simulink model "part1"  (R2023a)
settings: Solver=ode4  StartTime=0.0  StopTime=100  FixedStep=0.01  RelTol=1e-3
values from neighbouring files (symbols this model uses):
  Af = diag ([1/t1, 1/t2, 1/t3])    [init.m]
  Gamma_Matrix = diag(omega.^2)    [init.m]
  Kd = [2030000 5950000 763500000]    [init.m]
  Ki = [1586 23000 1068000]    [init.m]
  Kp = [114000 788000 78300000]    [init.m]
  Omega_Matrix = diag (2*zeta.*omega)    [init.m]
  P0 = eye(15)    [CPM.m]
  Q = eye(6)    [CPM.m]    (also in control_plant_model.m)
  R = eye(3)    [CPM.m]    (also in control_plant_model.m)
  ref_model = 1    [init.m]    (also in plotter.m; sim1.m; sim2.m; sim2_faulty.m)
  sample_time = 0.1    [CPM.m]    (also in init.m = 0.01)
  simulation = 4    [init.m]    (also in plotter.m)
  x0 = zeros(15,1)    [CPM.m]
undefined symbols (not defined in the file or in its folder): Hoerner, model, thrusters, vessel
libraries: eeStairGenerator x6, simulink x3, marine_gnc x3, slpidlib x3, marine_hydro x2
settings Model: Creator=jonbjor  LastModifiedBy=33769
settings SolverCC: AlgebraicLoopSolver=TrustRegion
settings DataIOCC: ReturnWorkspaceOutputs=off
settings DebuggingCC: UnconnectedInputMsg=warning  UnconnectedOutputMsg=warning  UnconnectedLineMsg=warning  ArithmeticOperatorsInVariantConditions=warning
settings ModelReferenceCC: EnableRefExpFcnMdlSchedulingChecks=on
settings SFSimCC: SimUseLocalCustomCode=off  CustomCodeUndefinedFunction=UseInterfaceOnly
settings RTWCC: RTWUseLocalCustomCode=off  DLArmComputeVersion=19.05

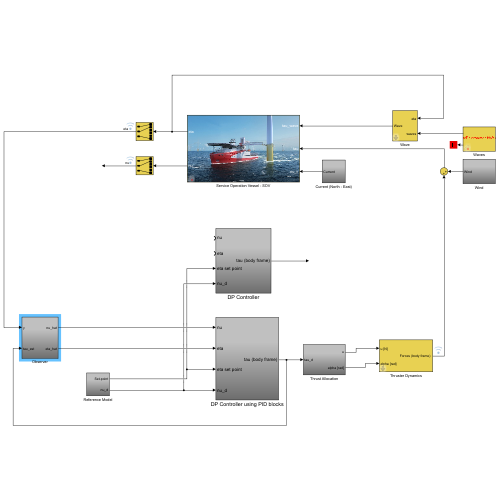
[thumbnail: Simulink's stored preview of the top-level diagram]
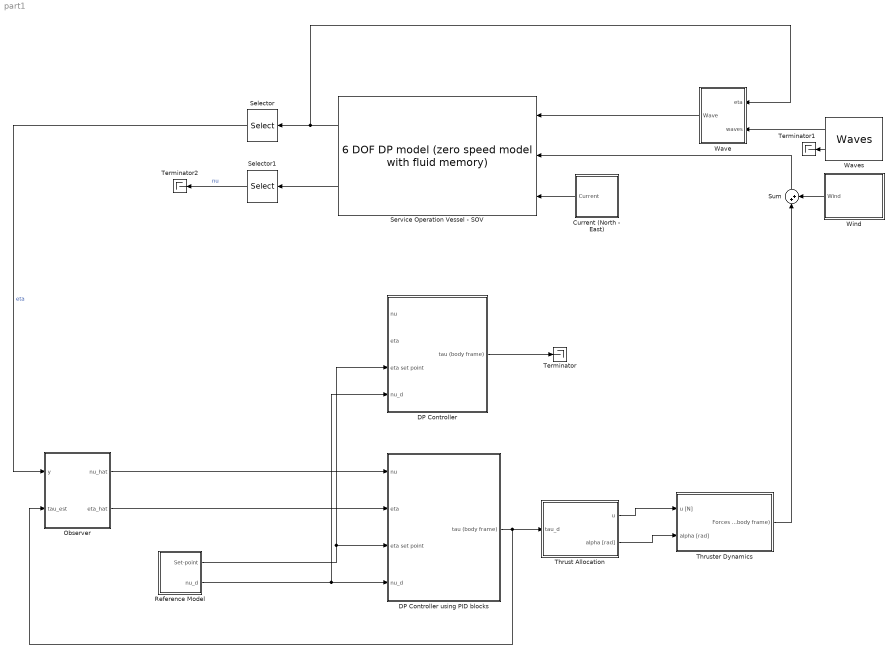
== system part1 ==
  Current (North - East) : Subsystem
  DP Controller : Subsystem
  DP Controller using PID blocks : Subsystem
  Observer : Subsystem
  Reference Model : Subsystem
  Selector : Selector  InputPortWidth=6  IndexOptions=Index vector (dialog)  Indices=[1 2 6]  OutputSizes=1
  Selector1 : Selector  InputPortWidth=6  IndexOptions=Index vector (dialog)  Indices=[1 2 6]  OutputSizes=1
  Service Operation Vessel - SOV : marine_hydro/Hydro Library/6 DOF DP model  (zero speed model with fluid memory)  ABC=vesselABC  rho=1025  Axc=0.9*vessel.main.T*vessel.main.B  Ayc=0.9*vessel.main.T*vessel.main.Lpp  CX=1  CY_2D=Hoerner(vessel.main.B,vessel.main.T)  Bv=vessel.Bv  mask(6 DOF zero speed model){}
      link override "Integrator1 ": InitialCondition=nu0
      link override Integrator2: InitialCondition=eta0
      mask Display:
      | image('SOV.jpg');
      | color('white'); port_label('output', 1, 'eta')
      | color('white'); port_label('output', 2, 'nu')
      | color('white'); port_label('input', 1, 'tau_wave')
      | color('white'); port_label('input', 2, 'tau')
      | color('white'); port_label('input', 3, 'nu_c')
  Sum : Sum  Inputs=|++
  Terminator : Terminator
  Terminator1 : Terminator
  Terminator2 : Terminator
  Thrust Allocation : Subsystem
  Thruster Dynamics : Subsystem  mask{thrusterfault=off}
      mask prompts: thrusterfault "Fault on thruster #2 and #4?"
  Wave : Subsystem  mask{waveforces=on}
      mask prompts: waveforces "Waveforces enabled"
  Waves : marine_gnc/Environment/Waves/Waves  spectrum_type=ITTC  disp_flag=on  plot_spectrum=off  plot_realization=off  hs=5  omega_peak=pi/10  psi_mean=0  gamma=-1  spread=2  depth=inf  nfreq=20  ndir=10  energylim=0.005  freq_cutoff=3  dir_cutoff=0  rand_seed=123  rand_freq=on  rand_dir=on  Zeta_a=0  Omega=0  Phase=0  Wavenum=0  Psi=0
  Wind : Subsystem
  wires:
  Current (North - East)/1(Current) -> Service Operation Vessel - SOV/3
  Service Operation Vessel - SOV/2 -> Selector1/1
  Selector/1 -> Observer/1(y)  "eta"
  Wave/1(Wave) -> Service Operation Vessel - SOV/1
  Reference Model/1(Set-point) -> DP Controller/3(eta set point), DP Controller using PID blocks/3(eta set point)
  Reference Model/2(nu_d) -> DP Controller/4(nu_d), DP Controller using PID blocks/4(nu_d)
  DP Controller/1(tau (body frame)) -> Terminator/1
  Waves/2 -> Terminator1/1
  Thruster Dynamics/1("Forces (body frame) ") -> Sum/1
  Service Operation Vessel - SOV/1 -> Wave/1(eta), Selector/1
  Wind/1(Wind) -> Sum/2
  Waves/1 -> Wave/2(waves)
  Sum/1 -> Service Operation Vessel - SOV/2
  Thrust Allocation/1(u) -> Thruster Dynamics/1(u [N])
  Thrust Allocation/2(alpha [rad]) -> Thruster Dynamics/2(alpha [rad])
  DP Controller using PID blocks/1(tau (body frame)) -> Observer/2(tau_est), Thrust Allocation/1(tau_d)
  Selector1/1 -> Terminator2/1  "nu"
  Observer/1(nu_hat) -> DP Controller using PID blocks/1(nu)
  Observer/2(eta_hat) -> DP Controller using PID blocks/2(eta)

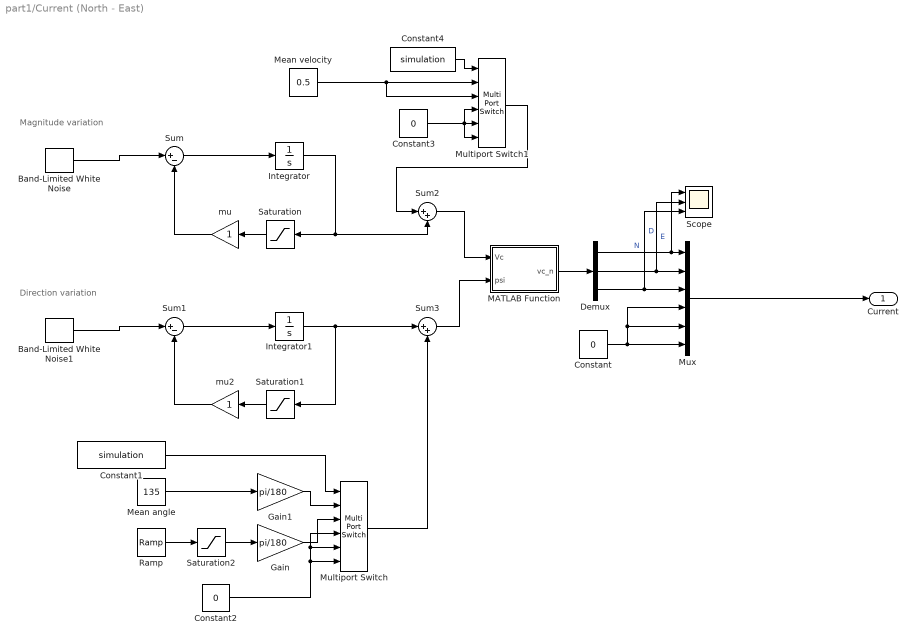
== system part1/Current (North - East) ==
  note: Magnitude variation
  note: Direction variation
  Band-Limited White Noise : simulink/Sources/Band-Limited White Noise  Cov=[0]  Ts=0.1  seed=[23341]
  Band-Limited White Noise1 : simulink/Sources/Band-Limited White Noise  Cov=[0]  Ts=0.1  seed=[23341]
  Constant : Constant  Value=0
  Constant1 : Constant  Value=simulation
  Constant2 : Constant  Value=0
  Constant3 : Constant  Value=0
  Constant4 : Constant  Value=simulation
  Demux : Demux  Outputs=3
  Gain : Gain  Gain=pi/180
  Gain1 : Gain  Gain=pi/180
  Integrator : Integrator
  Integrator1 : Integrator
  MATLAB Function : MATLAB Function  TreatAsAtomicUnit=on
  Mean angle : Constant  Value=135
  Mean velocity : Constant  Value=0.5
  Multiport Switch : MultiPortSwitch  Inputs=4  DataPortForDefault=Additional data port  SaturateOnIntegerOverflow=off  InputSameDT=off
  Multiport Switch1 : MultiPortSwitch  Inputs=4  DataPortForDefault=Additional data port  SaturateOnIntegerOverflow=off  InputSameDT=off
  Mux : Mux  Inputs=6
  Ramp : simulink/Sources/Ramp  slope=1  start=10  InitialOutput=180
  Saturation : Saturate  UpperLimit=1  LowerLimit=0
  Saturation1 : Saturate  UpperLimit=pi  LowerLimit=0
  Saturation2 : Saturate  UpperLimit=270  LowerLimit=0
  Scope : Scope  NumInputPorts=3
  Sum : Sum  Inputs=|+-
  Sum1 : Sum  Inputs=|+-
  Sum2 : Sum  Inputs=|++
  Sum3 : Sum  Inputs=|++
  mu : Gain
  mu2 : Gain
  Current : Outport  VectorParamsAs1DForOutWhenUnconnected=off
  wires:
  Band-Limited White Noise1/1 -> Sum1/1
  Mean velocity/1 -> Multiport Switch1/3, Multiport Switch1/2
  Mean angle/1 -> Gain1/1
  Saturation1/1 -> mu2/1
  Sum/1 -> Integrator/1
  Saturation2/1 -> Gain/1
  mu/1 -> Sum/2
  Constant3/1 -> Multiport Switch1/4, Multiport Switch1/6, Multiport Switch1/5
  Ramp/1 -> Saturation2/1
  Constant2/1 -> Multiport Switch/6, Multiport Switch/5, Multiport Switch/4
  Integrator1/1 -> Saturation1/1, Sum3/1
  Sum3/1 -> MATLAB Function/2(psi)
  Integrator/1 -> Sum2/2, Saturation/1
  Sum2/1 -> MATLAB Function/1(Vc)
  Multiport Switch1/1 -> Sum2/1
  MATLAB Function/1(vc_n) -> Demux/1
  Demux/1 -> Scope/1, Mux/1  "N"
  Constant/1 -> Mux/6, Mux/5, Mux/4
  mu2/1 -> Sum1/2
  Saturation/1 -> mu/1
  Demux/3 -> Scope/3, Mux/3  "D"
  Demux/2 -> Scope/2, Mux/2  "E"
  Gain/1 -> Multiport Switch/3
  Constant1/1 -> Multiport Switch/1
  Gain1/1 -> Multiport Switch/2
  Multiport Switch/1 -> Sum3/2
  Band-Limited White Noise/1 -> Sum/1
  Sum1/1 -> Integrator1/1
  Constant4/1 -> Multiport Switch1/1
  Mux/1 -> Current/1

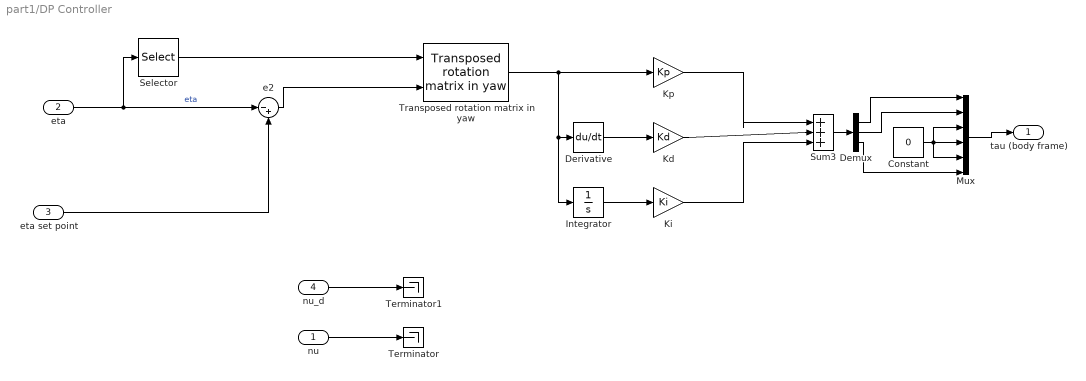
== system part1/DP Controller ==
  nu : Inport
  eta : Inport  Port=2
  eta set point : Inport  Port=3
  nu_d : Inport  Port=4
  Constant : Constant  Value=0
  Demux : Demux  Outputs=3
  Derivative : Derivative
  Integrator : Integrator
  Kd : Gain  Gain=Kd
  Ki : Gain  Gain=Ki
  Kp : Gain  Gain=Kp
  Mux : Mux  Inputs=6
  Selector : Selector  InputPortWidth=3  IndexOptions=Index vector (dialog)  Indices=3  OutputSizes=1
  Sum3 : Sum  Inputs=|+++
  Terminator : Terminator
  Terminator1 : Terminator
  Transposed rotation matrix in yaw : marine_gnc/Models/ Kinematics/Transposed rotation  matrix in yaw
  e2 : Sum  Inputs=|-+
  tau (body frame) : Outport  VectorParamsAs1DForOutWhenUnconnected=off
  wires:
  nu/1 -> Terminator/1
  e2/1 -> Transposed rotation matrix in yaw/2
  Transposed rotation matrix in yaw/1 -> Integrator/1, Derivative/1, Kp/1
  Kp/1 -> Sum3/1
  Derivative/1 -> Kd/1
  Kd/1 -> Sum3/2
  Integrator/1 -> Ki/1
  Ki/1 -> Sum3/3
  nu_d/1 -> Terminator1/1
  eta/1 -> Selector/1, e2/1  "eta"
  eta set point/1 -> e2/2
  Selector/1 -> Transposed rotation matrix in yaw/1
  Sum3/1 -> Demux/1
  Mux/1 -> tau (body frame)/1
  Demux/1 -> Mux/1
  Demux/2 -> Mux/2
  Demux/3 -> Mux/6
  Constant/1 -> Mux/5, Mux/4, Mux/3

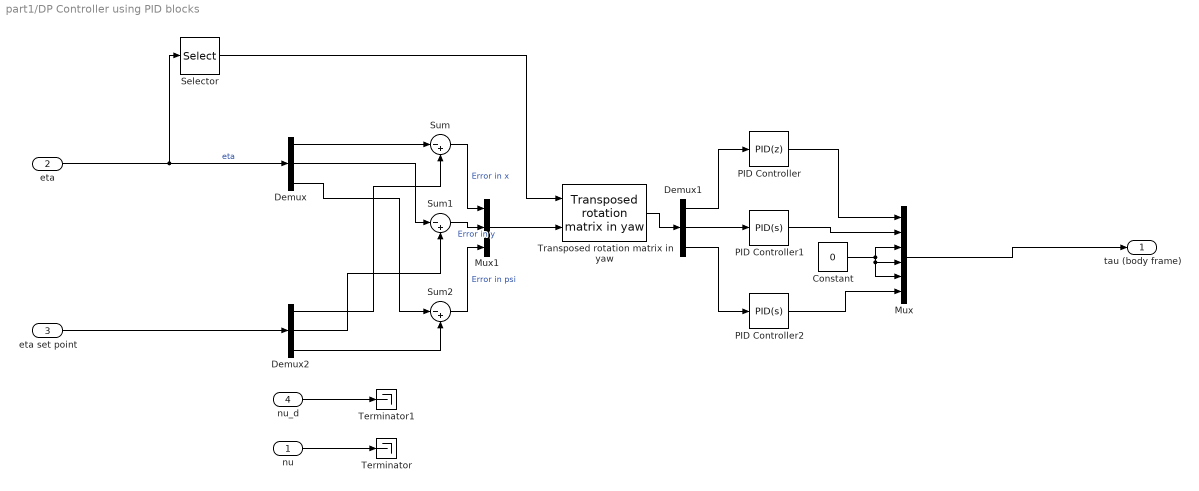
== system part1/DP Controller using PID blocks ==
  nu : Inport
  eta : Inport  Port=2
  eta set point : Inport  Port=3
  nu_d : Inport  Port=4
  Constant : Constant  Value=0
  Demux : Demux  Outputs=3
  Demux1 : Demux  Outputs=3
  Demux2 : Demux  Outputs=3
  Mux : Mux  Inputs=6
  Mux1 : Mux  Inputs=3
  PID Controller : slpidlib/PID Controller  Controller=PID  Form=Parallel  TimeDomain=Discrete-time  UseExternalTs=off  SampleTime=-1  IntegratorMethod=Forward Euler  FilterMethod=Forward Euler  ControllerParametersSource=internal  P=227096.416129913  I=4612.68202494015  UseKiTs=off  D=2289100.523399  N=34.1818873102708  UseFilter=on  TunerSelectOption=Transfer Function Based (PID Tuner App)  InitialConditionSource=internal  InitialConditionForIntegrator=0  InitialConditionForFilter=0  DifferentiatorICPrevScaledInput=0  ExternalReset=none  TrackingMode=off  Kt=1  LimitOutput=off  SatLimitsSource=internal  UpperSaturationLimit=inf  LowerSaturationLimit=-inf  LinearizeAsGain=on  AntiWindupMode=none  Kb=1  LimitIntegrator=off  UpperIntegratorSaturationLimit=inf  LowerIntegratorSaturationLimit=-inf  POutMin=[]  POutMax=[]  IOutMin=[]  IOutMax=[]  DOutMin=[]  DOutMax=[]  NOutMin=[]  NOutMax=[]  SumOutMin=[]  SumOutMax=[]  SaturationOutMin=[]  SaturationOutMax=[]  PParamMin=[]  PParamMax=[]  IParamMin=[]  IParamMax=[]  DParamMin=[]  DParamMax=[]  NParamMin=[]  NParamMax=[]  KbParamMin=[]  KbParamMax=[]  KtParamMin=[]  KtParamMax=[]  KbOutMin=[]  KbOutMax=[]  KtOutMin=[]  KtOutMax=[]  IntegratorOutMin=[]  IntegratorOutMax=[]  FilterOutMin=[]  FilterOutMax=[]  SumI1OutMin=[]  SumI1OutMax=[]  SumI2OutMin=[]  SumI2OutMax=[]  SumI3OutMin=[]  SumI3OutMax=[]  SumI4OutMin=[]  SumI4OutMax=[]  SumDOutMin=[]  SumDOutMax=[]  DifferentiatorOutMin=[]  DifferentiatorOutMax=[]  FilterDiffOutCoefMin=[]  FilterDiffOutCoefMax=[]  ReciprocalOutMin=[]  ReciprocalOutMax=[]  SumDenOutMin=[]  SumDenOutMax=[]  SumNumOutMin=[]  SumNumOutMax=[]  DivideOutMin=[]  DivideOutMax=[]  UdiffTsProdOutMin=[]  UdiffTsProdOutMax=[]  NTsProdOutMin=[]  NTsProdOutMax=[]  UintegralTsProdOutMin=[]  UintegralTsProdOutMax=[]  UngainTsProdOutMin=[]  UngainTsProdOutMax=[]  ClampingZeroOutDataTypeStr=Inherit: Inherit via back propagation  ClampingZeroOutMin=[]  ClampingZeroOutMax=[]  FilterDenConstantOutDataTypeStr=Inherit: Inherit via back propagation  FilterDenConstantOutMin=[]  FilterDenConstantOutMax=[]  PCopyOutDataTypeStr=Inherit: Inherit via back propagation  PCopyOutMin=[]  PCopyOutMax=[]  NCopyOutDataTypeStr=Inherit: Inherit via back propagation  NCopyOutMin=[]  NCopyOutMax=[]  IntegratorContinuousStateAttributes=''  IntegratorStateMustResolveToSignalObject=off  IntegratorRTWStateStorageClass=Auto  FilterContinuousStateAttributes=''  FilterStateMustResolveToSignalObject=off  FilterRTWStateStorageClass=Auto  ParallelPVariant=InternalParameters  IdealPVariant=Disabled  IVariant=InternalParameters  DVariant=InternalParameters  IntegratorVariant=Discrete  SatVariant=Disabled  AWVariant=Passthrough  PCopyVariant=Disabled  TRVariant=Disabled  FdbkBlocksVariant=Forward  IdealPFdbkVariant=Disabled  SatFdbkVariant=Disabled  DerivativeFilterVariant=ForwardEulerFilter  NVariant=InternalParameters  NCopyVariant=Disabled  FilterICVariant=InternalICsFilter  IntegratorICVariant=InternalICs  ExternalResetVariant=Disabled  TRSumVariant=Passthrough  SumFdbkVariant=Disabled  SumVariant=Sum_PID  TsampFilterVariant=InternalTs  TsampNgainVariant=Passthrough  TsampIntegralVariant=Disabled_SignalSpec  ExternalSaturationOutDataTypeStr=Inherit: Same as second input
  PID Controller1 : slpidlib/PID Controller  Controller=PID  Form=Parallel  TimeDomain=Continuous-time  UseExternalTs=off  SampleTime=-1  IntegratorMethod=Forward Euler  FilterMethod=Forward Euler  ControllerParametersSource=internal  P=1  I=1  UseKiTs=off  D=0  N=100  UseFilter=on  TunerSelectOption=Transfer Function Based (PID Tuner App)  InitialConditionSource=internal  InitialConditionForIntegrator=0  InitialConditionForFilter=0  DifferentiatorICPrevScaledInput=0  ExternalReset=none  TrackingMode=off  Kt=1  LimitOutput=off  SatLimitsSource=internal  UpperSaturationLimit=inf  LowerSaturationLimit=-inf  LinearizeAsGain=on  AntiWindupMode=none  Kb=1  LimitIntegrator=off  UpperIntegratorSaturationLimit=inf  LowerIntegratorSaturationLimit=-inf  POutMin=[]  POutMax=[]  IOutMin=[]  IOutMax=[]  DOutMin=[]  DOutMax=[]  NOutMin=[]  NOutMax=[]  SumOutMin=[]  SumOutMax=[]  SaturationOutMin=[]  SaturationOutMax=[]  PParamMin=[]  PParamMax=[]  IParamMin=[]  IParamMax=[]  DParamMin=[]  DParamMax=[]  NParamMin=[]  NParamMax=[]  KbParamMin=[]  KbParamMax=[]  KtParamMin=[]  KtParamMax=[]  KbOutMin=[]  KbOutMax=[]  KtOutMin=[]  KtOutMax=[]  IntegratorOutMin=[]  IntegratorOutMax=[]  FilterOutMin=[]  FilterOutMax=[]  SumI1OutMin=[]  SumI1OutMax=[]  SumI2OutMin=[]  SumI2OutMax=[]  SumI3OutMin=[]  SumI3OutMax=[]  SumI4OutMin=[]  SumI4OutMax=[]  SumDOutMin=[]  SumDOutMax=[]  DifferentiatorOutMin=[]  DifferentiatorOutMax=[]  FilterDiffOutCoefMin=[]  FilterDiffOutCoefMax=[]  ReciprocalOutMin=[]  ReciprocalOutMax=[]  SumDenOutMin=[]  SumDenOutMax=[]  SumNumOutMin=[]  SumNumOutMax=[]  DivideOutMin=[]  DivideOutMax=[]  UdiffTsProdOutMin=[]  UdiffTsProdOutMax=[]  NTsProdOutMin=[]  NTsProdOutMax=[]  UintegralTsProdOutMin=[]  UintegralTsProdOutMax=[]  UngainTsProdOutMin=[]  UngainTsProdOutMax=[]  ClampingZeroOutDataTypeStr=Inherit: Inherit via back propagation  ClampingZeroOutMin=[]  ClampingZeroOutMax=[]  FilterDenConstantOutDataTypeStr=Inherit: Inherit via back propagation  FilterDenConstantOutMin=[]  FilterDenConstantOutMax=[]  PCopyOutDataTypeStr=Inherit: Inherit via back propagation  PCopyOutMin=[]  PCopyOutMax=[]  NCopyOutDataTypeStr=Inherit: Inherit via back propagation  NCopyOutMin=[]  NCopyOutMax=[]  IntegratorContinuousStateAttributes=''  IntegratorStateMustResolveToSignalObject=off  IntegratorRTWStateStorageClass=Auto  FilterContinuousStateAttributes=''  FilterStateMustResolveToSignalObject=off  FilterRTWStateStorageClass=Auto  ParallelPVariant=InternalParameters  IdealPVariant=Disabled  IVariant=InternalParameters  DVariant=InternalParameters  IntegratorVariant=Continuous  SatVariant=Disabled  AWVariant=Passthrough  PCopyVariant=Disabled  TRVariant=Disabled  FdbkBlocksVariant=Forward  IdealPFdbkVariant=Disabled  SatFdbkVariant=Disabled  DerivativeFilterVariant=ContFilter  NVariant=InternalParameters  NCopyVariant=Disabled  FilterICVariant=InternalICsFilter  IntegratorICVariant=InternalICs  ExternalResetVariant=Disabled  TRSumVariant=Passthrough  SumFdbkVariant=Disabled  SumVariant=Sum_PID  TsampFilterVariant=InternalTs  TsampNgainVariant=Passthrough  TsampIntegralVariant=Disabled_SignalSpec  ExternalSaturationOutDataTypeStr=Inherit: Same as second input
  PID Controller2 : slpidlib/PID Controller  Controller=PID  Form=Parallel  TimeDomain=Continuous-time  UseExternalTs=off  SampleTime=-1  IntegratorMethod=Forward Euler  FilterMethod=Forward Euler  ControllerParametersSource=internal  P=1  I=1  UseKiTs=off  D=0  N=100  UseFilter=on  TunerSelectOption=Transfer Function Based (PID Tuner App)  InitialConditionSource=internal  InitialConditionForIntegrator=0  InitialConditionForFilter=0  DifferentiatorICPrevScaledInput=0  ExternalReset=none  TrackingMode=off  Kt=1  LimitOutput=off  SatLimitsSource=internal  UpperSaturationLimit=inf  LowerSaturationLimit=-inf  LinearizeAsGain=on  AntiWindupMode=none  Kb=1  LimitIntegrator=off  UpperIntegratorSaturationLimit=inf  LowerIntegratorSaturationLimit=-inf  POutMin=[]  POutMax=[]  IOutMin=[]  IOutMax=[]  DOutMin=[]  DOutMax=[]  NOutMin=[]  NOutMax=[]  SumOutMin=[]  SumOutMax=[]  SaturationOutMin=[]  SaturationOutMax=[]  PParamMin=[]  PParamMax=[]  IParamMin=[]  IParamMax=[]  DParamMin=[]  DParamMax=[]  NParamMin=[]  NParamMax=[]  KbParamMin=[]  KbParamMax=[]  KtParamMin=[]  KtParamMax=[]  KbOutMin=[]  KbOutMax=[]  KtOutMin=[]  KtOutMax=[]  IntegratorOutMin=[]  IntegratorOutMax=[]  FilterOutMin=[]  FilterOutMax=[]  SumI1OutMin=[]  SumI1OutMax=[]  SumI2OutMin=[]  SumI2OutMax=[]  SumI3OutMin=[]  SumI3OutMax=[]  SumI4OutMin=[]  SumI4OutMax=[]  SumDOutMin=[]  SumDOutMax=[]  DifferentiatorOutMin=[]  DifferentiatorOutMax=[]  FilterDiffOutCoefMin=[]  FilterDiffOutCoefMax=[]  ReciprocalOutMin=[]  ReciprocalOutMax=[]  SumDenOutMin=[]  SumDenOutMax=[]  SumNumOutMin=[]  SumNumOutMax=[]  DivideOutMin=[]  DivideOutMax=[]  UdiffTsProdOutMin=[]  UdiffTsProdOutMax=[]  NTsProdOutMin=[]  NTsProdOutMax=[]  UintegralTsProdOutMin=[]  UintegralTsProdOutMax=[]  UngainTsProdOutMin=[]  UngainTsProdOutMax=[]  ClampingZeroOutDataTypeStr=Inherit: Inherit via back propagation  ClampingZeroOutMin=[]  ClampingZeroOutMax=[]  FilterDenConstantOutDataTypeStr=Inherit: Inherit via back propagation  FilterDenConstantOutMin=[]  FilterDenConstantOutMax=[]  PCopyOutDataTypeStr=Inherit: Inherit via back propagation  PCopyOutMin=[]  PCopyOutMax=[]  NCopyOutDataTypeStr=Inherit: Inherit via back propagation  NCopyOutMin=[]  NCopyOutMax=[]  IntegratorContinuousStateAttributes=''  IntegratorStateMustResolveToSignalObject=off  IntegratorRTWStateStorageClass=Auto  FilterContinuousStateAttributes=''  FilterStateMustResolveToSignalObject=off  FilterRTWStateStorageClass=Auto  ParallelPVariant=InternalParameters  IdealPVariant=Disabled  IVariant=InternalParameters  DVariant=InternalParameters  IntegratorVariant=Continuous  SatVariant=Disabled  AWVariant=Passthrough  PCopyVariant=Disabled  TRVariant=Disabled  FdbkBlocksVariant=Forward  IdealPFdbkVariant=Disabled  SatFdbkVariant=Disabled  DerivativeFilterVariant=ContFilter  NVariant=InternalParameters  NCopyVariant=Disabled  FilterICVariant=InternalICsFilter  IntegratorICVariant=InternalICs  ExternalResetVariant=Disabled  TRSumVariant=Passthrough  SumFdbkVariant=Disabled  SumVariant=Sum_PID  TsampFilterVariant=InternalTs  TsampNgainVariant=Passthrough  TsampIntegralVariant=Disabled_SignalSpec  ExternalSaturationOutDataTypeStr=Inherit: Same as second input
  Selector : Selector  InputPortWidth=3  IndexOptions=Index vector (dialog)  Indices=3  OutputSizes=1
  Sum : Sum  Inputs=|-+
  Sum1 : Sum  Inputs=|-+
  Sum2 : Sum  Inputs=|-+
  Terminator : Terminator
  Terminator1 : Terminator
  Transposed rotation matrix in yaw : marine_gnc/Models/ Kinematics/Transposed rotation  matrix in yaw
  tau (body frame) : Outport  VectorParamsAs1DForOutWhenUnconnected=off
  wires:
  nu_d/1 -> Terminator1/1
  Mux/1 -> tau (body frame)/1
  Constant/1 -> Mux/3, Mux/4, Mux/5
  PID Controller2/1 -> Mux/6
  nu/1 -> Terminator/1
  PID Controller1/1 -> Mux/2
  PID Controller/1 -> Mux/1
  Demux2/3 -> Sum2/2
  Demux/3 -> Sum2/1
  Demux2/2 -> Sum1/2
  Demux/2 -> Sum1/1
  Demux2/1 -> Sum/2
  Demux/1 -> Sum/1
  eta set point/1 -> Demux2/1
  eta/1 -> Selector/1, Demux/1  "eta"
  Sum/1 -> Mux1/1  "Error in x"
  Sum1/1 -> Mux1/2  "Error in y"
  Sum2/1 -> Mux1/3  "Error in psi"
  Mux1/1 -> Transposed rotation matrix in yaw/2
  Selector/1 -> Transposed rotation matrix in yaw/1
  Transposed rotation matrix in yaw/1 -> Demux1/1
  Demux1/1 -> PID Controller/1
  Demux1/2 -> PID Controller1/1
  Demux1/3 -> PID Controller2/1

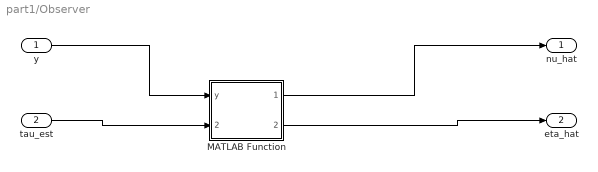
== system part1/Observer ==
  y : Inport
  tau_est : Inport  Port=2
  MATLAB Function : MATLAB Function  TreatAsAtomicUnit=on
  nu_hat : Outport  VectorParamsAs1DForOutWhenUnconnected=off
  eta_hat : Outport  Port=2  VectorParamsAs1DForOutWhenUnconnected=off
  wires:
  y/1 -> MATLAB Function/1(y)
  tau_est/1 -> MATLAB Function/2(tau_est)
  MATLAB Function/1(nu_hat) -> nu_hat/1
  MATLAB Function/2(eta_hat) -> eta_hat/1

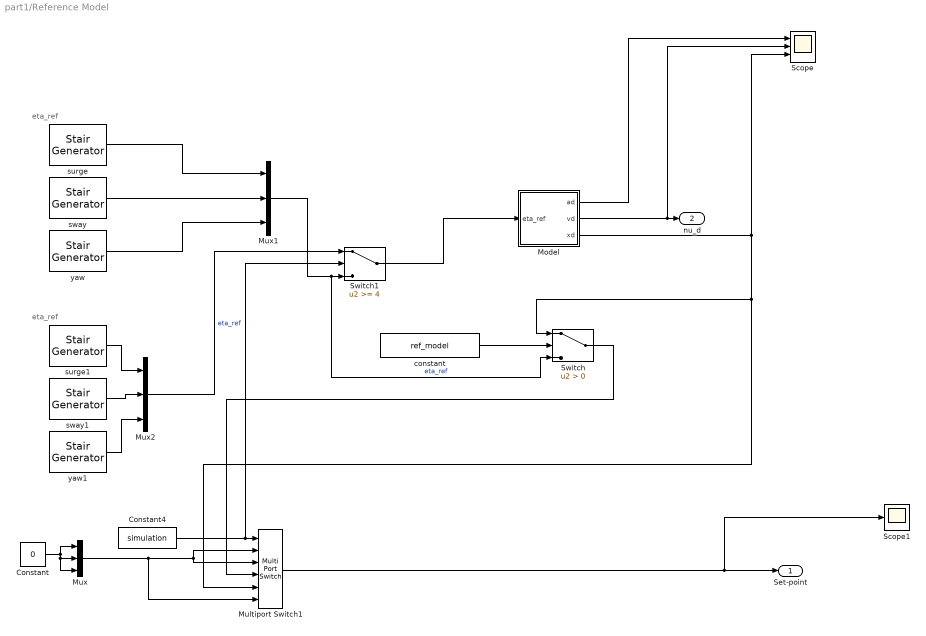
== system part1/Reference Model ==
  note: eta_ref
  note: eta_ref
  Constant : Constant  Value=0
  Constant4 : Constant  Value=simulation
  Model : Subsystem
  Multiport Switch1 : MultiPortSwitch  Inputs=4  DataPortForDefault=Additional data port  SaturateOnIntegerOverflow=off  InputSameDT=off
  Mux : Mux  Inputs=3
  Mux1 : Mux  Inputs=3
  Mux2 : Mux  Inputs=3
  Scope : Scope  NumInputPorts=3
  Scope1 : Scope
  Switch : Switch  Criteria=u2 > Threshold  SaturateOnIntegerOverflow=off  InputSameDT=off
  Switch1 : Switch  Threshold=4  SaturateOnIntegerOverflow=off  InputSameDT=off
  constant : Constant  Value=ref_model
  surge : eeStairGenerator/Stair Generator  LabelModeActiveChoice=Discrete  TimeInput=[10]  AmplitudeInput=[10]  SampleTime=sample_time  RepeatPattern=off  OutDataTypeStr=double
      settings: LibrarySourceBlock=ee_sl_lib/General Control/Stair Generator
  surge1 : eeStairGenerator/Stair Generator  LabelModeActiveChoice=Discrete  TimeInput=[100 200 300 400 500]  AmplitudeInput=[50 50 50 0 0 ]  SampleTime=sample_time  RepeatPattern=off  OutDataTypeStr=double
      settings: LibrarySourceBlock=ee_sl_lib/General Control/Stair Generator
  sway : eeStairGenerator/Stair Generator  LabelModeActiveChoice=Discrete  TimeInput=[10]  AmplitudeInput=[10]  SampleTime=sample_time  RepeatPattern=off  OutDataTypeStr=double
      settings: LibrarySourceBlock=ee_sl_lib/General Control/Stair Generator
  sway1 : eeStairGenerator/Stair Generator  LabelModeActiveChoice=Discrete  TimeInput=[100 200 300 400 500]  AmplitudeInput=[0 -50 -50 -50 0]  SampleTime=sample_time  RepeatPattern=off  OutDataTypeStr=double
      settings: LibrarySourceBlock=ee_sl_lib/General Control/Stair Generator
  yaw : eeStairGenerator/Stair Generator  LabelModeActiveChoice=Discrete  TimeInput=[10]  AmplitudeInput=[3*pi/2]  SampleTime=sample_time  RepeatPattern=off  OutDataTypeStr=double
      settings: LibrarySourceBlock=ee_sl_lib/General Control/Stair Generator
  yaw1 : eeStairGenerator/Stair Generator  LabelModeActiveChoice=Discrete  TimeInput=[100 200 300 400 500]  AmplitudeInput=[0 0 -pi/4 -pi/4 0]  SampleTime=sample_time  RepeatPattern=off  OutDataTypeStr=double
      settings: LibrarySourceBlock=ee_sl_lib/General Control/Stair Generator
  Set-point : Outport  VectorParamsAs1DForOutWhenUnconnected=off
  nu_d : Outport  Port=2
  wires:
  sway/1 -> Mux1/2
  Model/1(ad) -> Scope/1
  yaw/1 -> Mux1/3
  Constant/1 -> Mux/1, Mux/3, Mux/2
  surge/1 -> Mux1/1
  sway1/1 -> Mux2/2
  Mux/1 -> Multiport Switch1/6, Multiport Switch1/2, Multiport Switch1/3
  Switch/1 -> Multiport Switch1/4
  yaw1/1 -> Mux2/3
  Switch1/1 -> Model/1(eta_ref)
  surge1/1 -> Mux2/1
  Mux1/1 -> Switch/3, Switch1/3  "eta_ref"
  Model/3(xd) -> Scope/3, Multiport Switch1/5, Switch/1
  constant/1 -> Switch/2
  Multiport Switch1/1 -> Scope1/1, Set-point/1
  Model/2(vd) -> Scope/2, nu_d/1
  Constant4/1 -> Switch1/2, Multiport Switch1/1
  Mux2/1 -> Switch1/1  "eta_ref"

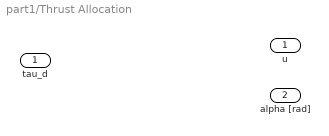
== system part1/Thrust Allocation ==
  tau_d : Inport
  u : Outport  VectorParamsAs1DForOutWhenUnconnected=off
  alpha [rad] : Outport  Port=2  VectorParamsAs1DForOutWhenUnconnected=off

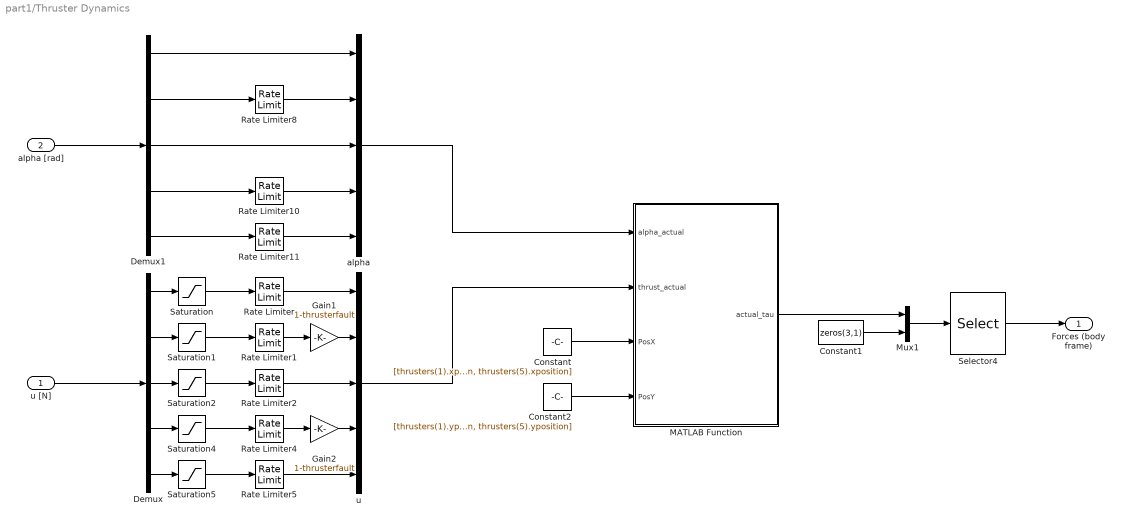
== system part1/Thruster Dynamics ==
  u [N] : Inport
  alpha [rad] : Inport  Port=2
  Constant : Constant  Value=[thrusters(1).xposition, thrusters(2).xposition, thrusters(3).xposition, thrusters(4).xposition, thrusters(5).xposition]
  Constant1 : Constant  Value=zeros(3,1)
  Constant2 : Constant  Value=[thrusters(1).yposition, thrusters(2).yposition, thrusters(3).yposition, thrusters(4).yposition, thrusters(5).yposition]
  Demux : Demux  Outputs=5
  Demux1 : Demux  Outputs=5
  Gain1 : Gain  Gain=1-thrusterfault
  Gain2 : Gain  Gain=1-thrusterfault
  MATLAB Function : MATLAB Function  TreatAsAtomicUnit=on
  Mux1 : Mux  Inputs=2
  Rate Limiter : RateLimiter  RisingSlewLimit=thrusters(1).rate  FallingSlewLimit=-thrusters(1).rate  SampleTimeMode=inherited
  Rate Limiter1 : RateLimiter  RisingSlewLimit=thrusters(2).rate  FallingSlewLimit=-thrusters(2).rate  SampleTimeMode=inherited
  Rate Limiter10 : RateLimiter  RisingSlewLimit=thrusters(4).rotationspeed  FallingSlewLimit=-thrusters(4).rotationspeed  SampleTimeMode=inherited
  Rate Limiter11 : RateLimiter  RisingSlewLimit=thrusters(5).rotationspeed  FallingSlewLimit=-thrusters(5).rotationspeed  SampleTimeMode=inherited
  Rate Limiter2 : RateLimiter  RisingSlewLimit=thrusters(3).rate  FallingSlewLimit=-thrusters(3).rate  SampleTimeMode=inherited
  Rate Limiter4 : RateLimiter  RisingSlewLimit=thrusters(4).rate  FallingSlewLimit=-thrusters(4).rate  SampleTimeMode=inherited
  Rate Limiter5 : RateLimiter  RisingSlewLimit=thrusters(5).rate  FallingSlewLimit=-thrusters(5).rate  SampleTimeMode=inherited
  Rate Limiter8 : RateLimiter  RisingSlewLimit=thrusters(2).rotationspeed  FallingSlewLimit=-thrusters(2).rotationspeed  SampleTimeMode=inherited
  Saturation : Saturate  UpperLimit=thrusters(1).thrust  LowerLimit=-thrusters(1).thrust
  Saturation1 : Saturate  UpperLimit=thrusters(2).thrust  LowerLimit=-thrusters(2).thrust
  Saturation2 : Saturate  UpperLimit=thrusters(3).thrust  LowerLimit=-thrusters(3).thrust
  Saturation4 : Saturate  UpperLimit=thrusters(4).thrust  LowerLimit=-thrusters(4).thrust
  Saturation5 : Saturate  UpperLimit=thrusters(5).thrust  LowerLimit=-thrusters(5).thrust
  Selector4 : Selector  InputPortWidth=6  IndexOptions=Index vector (dialog)  Indices=[1 2 4 5 6 3]  OutputSizes=1
  alpha : Mux  Inputs=5
  u : Mux  Inputs=5
  "Forces (body frame) " : Outport  VectorParamsAs1DForOutWhenUnconnected=off
  wires:
  Rate Limiter2/1 -> u/3
  Saturation/1 -> Rate Limiter/1
  Mux1/1 -> Selector4/1
  Constant1/1 -> Mux1/2
  Saturation4/1 -> Rate Limiter4/1
  Demux/2 -> Saturation1/1
  Saturation1/1 -> Rate Limiter1/1
  Demux/1 -> Saturation/1
  Demux/3 -> Saturation2/1
  Saturation2/1 -> Rate Limiter2/1
  Selector4/1 -> "Forces (body frame) "/1
  Gain1/1 -> u/2
  Rate Limiter1/1 -> Gain1/1
  Rate Limiter/1 -> u/1
  Rate Limiter4/1 -> Gain2/1
  Saturation5/1 -> Rate Limiter5/1
  u [N]/1 -> Demux/1
  alpha [rad]/1 -> Demux1/1
  Constant/1 -> MATLAB Function/3(PosX)
  Constant2/1 -> MATLAB Function/4(PosY)
  u/1 -> MATLAB Function/2(thrust_actual)
  alpha/1 -> MATLAB Function/1(alpha_actual)
  MATLAB Function/1(actual_tau) -> Mux1/1
  Rate Limiter10/1 -> alpha/4
  Demux1/4 -> Rate Limiter10/1
  Demux1/5 -> Rate Limiter11/1
  Rate Limiter11/1 -> alpha/5
  Demux1/1 -> alpha/1
  Gain2/1 -> u/4
  Demux/4 -> Saturation4/1
  Demux/5 -> Saturation5/1
  Rate Limiter5/1 -> u/5
  Demux1/2 -> Rate Limiter8/1
  Rate Limiter8/1 -> alpha/2
  Demux1/3 -> alpha/3

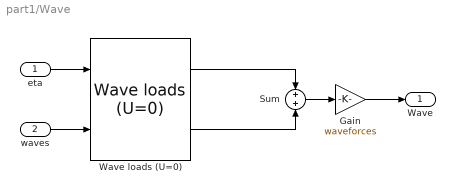
== system part1/Wave ==
  eta : Inport
  waves : Inport  Port=2
  Gain : Gain  Gain=waveforces
  Sum : Sum
  Wave loads (U=0) : marine_hydro/Hydro Library/Wave loads (U=0)  SystemSampleTime=-1  VariantActivationTime=update diagram  Latency=0  AutoFrameSizeCalculation=off
  Wave : Outport  VectorParamsAs1DForOutWhenUnconnected=off
  wires:
  eta/1 -> Wave loads (U=0)/1
  waves/1 -> Wave loads (U=0)/2
  Sum/1 -> Gain/1
  Wave loads (U=0)/1 -> Sum/1
  Wave loads (U=0)/2 -> Sum/2
  Gain/1 -> Wave/1

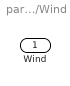
== system part1/Wind ==
  Wind : Outport  VectorParamsAs1DForOutWhenUnconnected=off

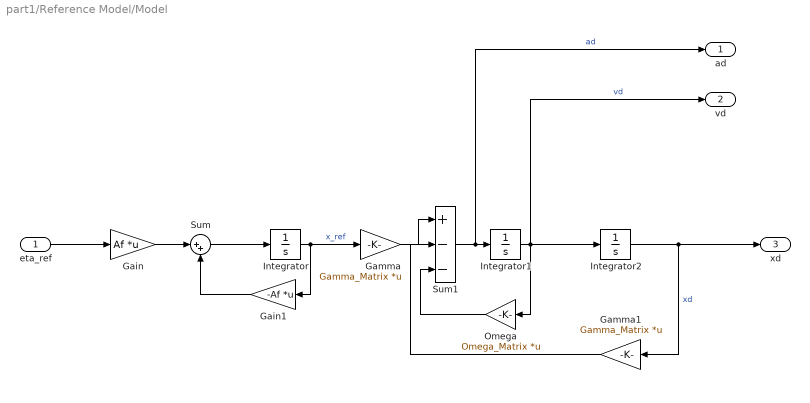
== system part1/Reference Model/Model ==
  eta_ref : Inport
  Gain : Gain  Gain=Af  Multiplication=Matrix(K*u)
  Gain1 : Gain  Gain=-Af  Multiplication=Matrix(K*u)
  Gamma : Gain  Gain=Gamma_Matrix  Multiplication=Matrix(K*u)
  Gamma1 : Gain  Gain=Gamma_Matrix  Multiplication=Matrix(K*u)
  Integrator : Integrator
  Integrator1 : Integrator
  Integrator2 : Integrator
  Omega : Gain  Gain=Omega_Matrix  Multiplication=Matrix(K*u)
  Sum : Sum  Inputs=|++
  Sum1 : Sum  Inputs=|+--
  ad : Outport
  vd : Outport  Port=2
  xd : Outport  Port=3
  wires:
  Omega/1 -> Sum1/3
  Integrator/1 -> Gamma/1, Gain1/1  "x_ref"
  Integrator1/1 -> Integrator2/1, Omega/1, vd/1  "vd"
  Gain/1 -> Sum/1
  Gamma1/1 -> Sum1/2
  Sum1/1 -> ad/1, Integrator1/1  "ad"
  Sum/1 -> Integrator/1
  Gamma/1 -> Sum1/1
  Integrator2/1 -> Gamma1/1, xd/1  "xd"
  Gain1/1 -> Sum/2
  eta_ref/1 -> Gain/1

== matlab function part1/Observer/MATLAB Function ==
  data: nu_hat output; eta_hat output; y input; tau_est input; sample_time parameter; model parameter; Q parameter; R parameter; x0 parameter; P0 parameter
function [nu_hat, eta_hat]= fcn(y,tau_est, sample_time, model, Q, R, x0, P0)
y_k = y;
%model
%x = [zeta eta bias nu]

%intailization
persistent x_k
persistent P_k
        
if isempty(x_k)
    x_k = x0;
end
if isempty (P_k)
    P_k = P0;
end

zeta = x_k(1:6); eta = x_k(7:9); b = x_k(10:12); nu = x_k(13:15);
u,v,r = nu;

%rotation matrix
psi = x_k(9);
c = cos(psi);
s = sin(psi);

% Create the rotation matrix R(ψ)
R_psi = [c, -s, 0;
     s, c, 0;
     0, 0, 1];

M_inv = model.M_inv;

f_x = [model.A_w * zeta;
        R_psi * nu;
        -inv(model.T_b) * b;
        -M_inv * model.D * nu + M_inv * R_psi' * b];

jac_f_x = [model.A_w zeros(3,3) zeros(3,3) zeros(3,3);
           zeros(3,6) zeros(3,3) zeros(3,3) R_psi;
           zeros(3,3) zeros(3,3) -inv(model.T_b) zeros(3,3);
           zeros(3,6) zeros(3,3) M_inv * R_psi' -M_inv * model.D];

%parial derivative of f_x with respect to psi
jac_f_x(7,9) = - sin(psi) * u - cos(psi) * v ;
jac_f_x(8,9) = cos(psi) * u - sin(psi) * v ;
jac_f_x(9,9) = 0 ;
diff_R = [-s -c 0;
          c -s 0;
          0 0 0]; 
jac_f_x(13:15,9) = M_inv * diff_R' * b ;

B = [zeros(6,3);
    zeros(3,3);
    zeros(3,3);
    M_inv];

E = [model.E_w zeros(6,3);
    zeros(3,3) zeros(3,3);
    zeros(3,3) model.E_b;
    zeros(3,3) zeros(3,3)];

H = [model.C_w eye(3) zeros(3,3) zeros(3,3)];

Phi_k = eye(model.n_states) + sample_time * jac_f_x;
Gamma_k = sample_time * E;

%Corrector
K_k = P_k * H' * (H * P_k * H')^(-1);
P_k_ = (eye(model.n_states) - K_k * H) * P_k * (eye(model.n_states) - K_k * H)' + K_k * R * K_k';
x_k_ = x_k + K_k * (y_k - H * x_k);

%predictor
P_k = Phi_k * P_k_ * Phi_k' + Gamma_k * Q * Gamma_k';
x_k = x_k_ + sample_time * (f_x + B * tau_est );

eta_hat = x_k_(7:9) ;
nu_hat = x_k_(13:15);

== matlab function part1/Current (North - East)/MATLAB Function ==
  data: Vc input; vc_n output; psi input
function vc_n = fcn(Vc, psi)


vc_n =[Vc * cos(psi);
     Vc * sin(psi);
     0];

== matlab function part1/Thruster Dynamics/MATLAB Function ==
  data: alpha_actual input; thrust_actual input; actual_tau output; PosX input; PosY input
function actual_tau   = fcn(alpha_actual,thrust_actual,PosX,PosY)

    Alpha_surge =[cos(alpha_actual(1)) cos(alpha_actual(2)) cos(alpha_actual(3)) cos(alpha_actual(4)) cos(alpha_actual(5))];  
    Alpha_sway = [sin(alpha_actual(1)) sin(alpha_actual(2)) sin(alpha_actual(3)) sin(alpha_actual(4)) sin(alpha_actual(5))];
    Alpha_yaw = [sin(alpha_actual(1))*PosX(1)-cos(alpha_actual(1))*PosY(1) sin(alpha_actual(2))*PosX(2)-cos(alpha_actual(2))*PosY(2) ...
                 sin(alpha_actual(3))*PosX(3)-cos(alpha_actual(3))*PosY(3) sin(alpha_actual(4))*PosX(4)-cos(alpha_actual(4))*PosY(4) ...
                 sin(alpha_actual(5))*PosX(5)-cos(alpha_actual(5))*PosY(5)];

    actual_tau = [Alpha_surge; Alpha_sway; Alpha_yaw]*thrust_actual;
end
